simulink model "LAB2_DirectDiscreteDesign_Robust"  (R2025b)
settings: Solver=VariableStepAuto  StartTime=0.0  StopTime=2  FixedStep=T  RelTol=1e-3
values from neighbouring files (symbols this model uses):
  gamma_o = [gamma(2)-L*gamma(1), (phi22-L*phi12)*L+phi21-L*phi11]    [LAB2_2_DDD_Robust.m]
  Ho = [0;1]    [LAB2_2_DDD_Robust.m]
  Jo = [0 1; 0 L]    [LAB2_2_DDD_Robust.m]
  K = Ke(2:3)    [LAB2_2_DDD_Robust.m]
  Ki = Ke(1)    [LAB2_2_DDD_Robust.m]
  Nr = Nu + K * Nx    [LAB2_2_DDD_Robust.m]
  phi_o = lambda_o_dt    [LAB2_2_DDD_Robust.m]
  step_amplitude = 60    [LAB2_2_DDD_Robust.m]
  T = 0.2    [LAB2_2_DDD_Robust.m]
undefined symbols (not defined in the file or in its folder): DiscIntNeverNeededParam, pulse2deg
settings Model: ExtModeTrigDuration=100001  Creator=delpratogi  LastModifiedBy=Gioele
settings HardwareCC: ProdBitPerLong=64.0  ProdHWDeviceType=Intel->x86-64 (Linux 64)
settings RTWCC: SystemTargetFile=sldrt.tlc  TemplateMakefile=sldrt.tmf  RTWCompilerOptimization=on  Description=Simulink Desktop Real-Time
settings CodeAppCC: MaxIdLength=95.0
settings SimulinkDesktopRealTimeCC: ExtModeTransport=0.0  ExtModeStaticAllocSize=1000000.0  TargetLibSuffix=_sldrt.a  TargetPreCompLibLocation=C:\Program Files\MATLAB\R2025b\toolbox\sldrt\lib\win64  MultiwordLength=2048.0  DynamicStringBufferSize=256.0  ParMdlRefBuildCompliant=on  PreserveMATLABNamespacesInGeneratedCode=on  SubcomponentCodeInterfacePackaging=Reusable function  SupportVariableSizeSignals=off

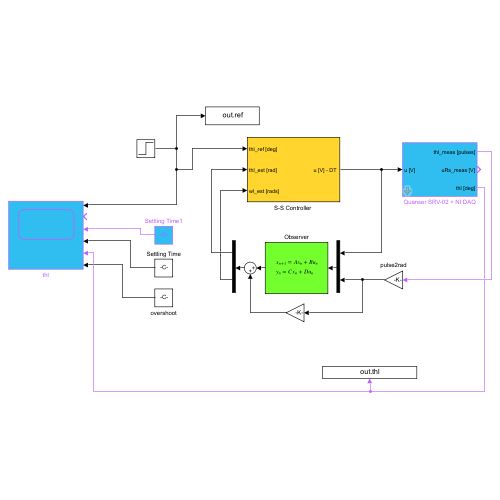
[thumbnail: Simulink's stored preview of the top-level diagram]
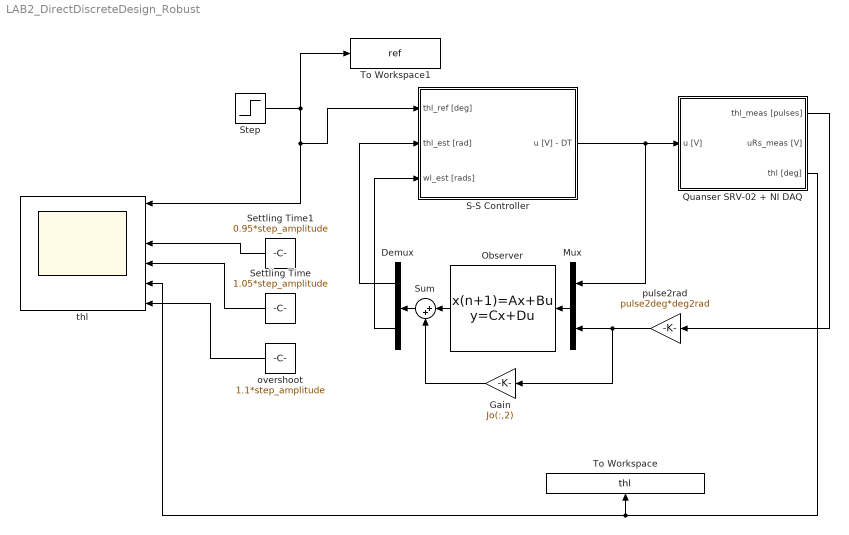
== system LAB2_DirectDiscreteDesign_Robust ==
  Demux : Demux  Outputs=2
  Gain : Gain  Gain=Jo(:,2)
  Mux : Mux  Inputs=2
  Observer : DiscreteStateSpace  A=phi_o  B=gamma_o  C=Ho  D=zeros(2,2)  SampleTime=T
  Quanser SRV-02 + NI DAQ : Subsystem  mask(Quanser SRV-02 (with inertial load) + NI DAQ){Ts=T, fricType=Coulomb + viscous}
      mask prompts: Ts "NI DAQ Sample Time:"; fricType "Friction model"
      mask help: Quanser SRV-02 (with inertial load) + NI DAQ model.
      mask init:
      | %%  Sensors data
      | 
      | %   shunt resistor
      | sens.curr.Rs = 0.5;                         %   resistance [Ohm]   
      | sens.curr.uRs_std = 0.01;                   %   voltage noise standard dev [V]                           
      | sens.curr.uRs_var = sens.curr.uRs_std^2;	%   voltage noise variance [V^2]
      | 
      | %   Hewlett-Packard HEDS-5540#A06 optical encoder
      | sens.enc.ppr = 500*4;                       %   pulses per rotation
      | sens.enc.pulse2deg = 360/sens.enc.ppr;      %   [pulses] -> [deg]
      | sens.enc.pulse2rad = 2*pi/sens.enc.ppr;     %   [pulses] -> [rad]
      | sens.enc.deg2pulse = sens.enc.ppr/360;      %   [deg] -> [pulses]
      | sens.enc.rad2pulse = sens.enc.ppr/2/pi;     %   [rad] -> [pulses]
      | 
      | 
      | %%  Data acquisition board (daq) data
      | 
      | %   NI PCI-6221 DAC data
      | daq.dac.bits = 16;                                  %   resolution (bits)
      | daq.dac.fs   = 10;                                  %   full scale 
      | daq.dac.q    = 2*daq.dac.fs/(2^daq.dac.bits-1);     %	quantization
      | 
      | %   NI PCI-6221 ADC data
      | daq.adc.bits = 16;                                  %   resolution (bits)
      | daq.adc.fs   = 10;                                  %   full scale (as set in SLDRT Analog Input block)
      | daq.adc.q    = 2*daq.adc.fs/(2^daq.adc.bits-1);     %   quantization
      mask Help:
      | Riccardo Antonello (antonello@dei.unipd.it)
      | 
      | April 24, 2020
      | 
      | Dept. of Information Engineering, University of Padova
      mask TypeOptions fricType: Coulomb + viscous | Karnopp
  "S-S Controller " : Subsystem
  Settling Time : Constant  Value=1.05*step_amplitude
  Settling Time1 : Constant  Value=0.95*step_amplitude
  Step : Step  Time=0  After=step_amplitude  ZeroCross=off
  Sum : Sum  Inputs=|++
  To Workspace : ToWorkspace  VariableName=thl  SaveFormat=Structure With Time  SampleTime=-1
  To Workspace1 : ToWorkspace  VariableName=ref  SaveFormat=Structure With Time  SampleTime=-1
  overshoot : Constant  Value=1.1*step_amplitude
  pulse2rad : Gain  Gain=pulse2deg*deg2rad
  thl : Scope  NumInputPorts=6
      settings: ActiveDisplayYMinimum=-8.2499999999999982  ActiveDisplayYMaximum=74.25
  wires:
  Demux/2 -> "S-S Controller "/3(wl_est [rads])
  "S-S Controller "/1("u [V] - DT ") -> Quanser SRV-02 + NI DAQ/1(u [V]), Mux/1
  Demux/1 -> "S-S Controller "/2(thl_est [rad])
  Mux/1 -> Observer/1
  Quanser SRV-02 + NI DAQ/1(thl_meas [pulses]) -> pulse2rad/1
  pulse2rad/1 -> Gain/1, Mux/2
  Sum/1 -> Demux/1
  Observer/1 -> Sum/1
  Gain/1 -> Sum/2
  overshoot/1 -> thl/6
  Settling Time/1 -> thl/4
  Settling Time1/1 -> thl/3
  Step/1 -> To Workspace1/1, thl/1, "S-S Controller "/1(thl_ref [deg])
  Quanser SRV-02 + NI DAQ/3(thl [deg]) -> thl/5, To Workspace/1

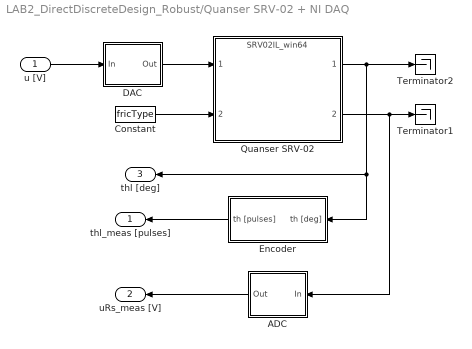
== system LAB2_DirectDiscreteDesign_Robust/Quanser SRV-02 + NI DAQ ==
  u [V] : Inport
  ADC : Subsystem
  Constant : Constant  Value=fricType
  DAC : Subsystem
  Encoder : Subsystem
  Quanser SRV-02 : ModelReference  ModelNameDialog=SRV02IL_win64.slxp  ModelReferenceVersion=1.44  CopyOfModelProtected=on
  Terminator1 : Terminator
  Terminator2 : Terminator
  thl_meas [pulses] : Outport
  uRs_meas [V] : Outport  Port=2
  thl [deg] : Outport  Port=3
  wires:
  Encoder/1(th [pulses]) -> thl_meas [pulses]/1
  ADC/1(Out) -> uRs_meas [V]/1
  DAC/1(Out) -> Quanser SRV-02/1
  Quanser SRV-02/2 -> ADC/1(In), Terminator1/1
  u [V]/1 -> DAC/1(In)
  Constant/1 -> Quanser SRV-02/2
  Quanser SRV-02/1 -> Encoder/1(th [deg]), thl [deg]/1, Terminator2/1

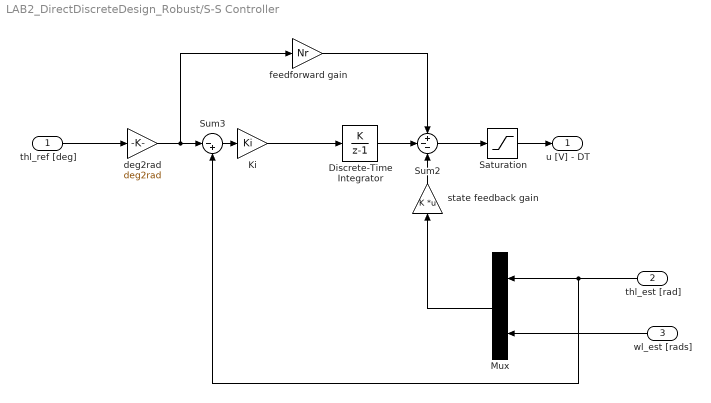
== system LAB2_DirectDiscreteDesign_Robust/S-S Controller  ==
  thl_ref [deg] : Inport
  thl_est [rad] : Inport  Port=2
  wl_est [rads] : Inport  Port=3
  " feedforward gain" : Gain  Gain=Nr
  Discrete-Time Integrator : DiscreteIntegrator  IntegratorMethod=Accumulation: Forward Euler  SampleTime=T  ICPrevOutput=DiscIntNeverNeededParam  ICPrevScaledInput=DiscIntNeverNeededParam
  Ki : Gain  Gain=Ki
  Mux : Mux  Inputs=2
  Saturation : Saturate  UpperLimit=10  LowerLimit=-10  ZeroCross=off
  Sum2 : Sum  Inputs=+--
  Sum3 : Sum  Inputs=|-+
  deg2rad : Gain  Gain=deg2rad
  state feedback gain : Gain  Gain=K  Multiplication=Matrix(K*u)
  "u [V] - DT " : Outport
  wires:
  Mux/1 -> state feedback gain/1
  deg2rad/1 -> " feedforward gain"/1, Sum3/1
  Sum2/1 -> Saturation/1
  Saturation/1 -> "u [V] - DT "/1
  thl_est [rad]/1 -> Sum3/2, Mux/1
  state feedback gain/1 -> Sum2/3
  " feedforward gain"/1 -> Sum2/1
  thl_ref [deg]/1 -> deg2rad/1
  wl_est [rads]/1 -> Mux/2
  Discrete-Time Integrator/1 -> Sum2/2
  Sum3/1 -> Ki/1
  Ki/1 -> Discrete-Time Integrator/1

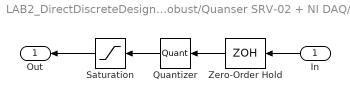
== system LAB2_DirectDiscreteDesign_Robust/Quanser SRV-02 + NI DAQ/ADC ==
  In : Inport
  Quantizer : Quantizer  QuantizationInterval=daq.adc.q
  Saturation : Saturate  UpperLimit=daq.adc.fs  LowerLimit=-daq.adc.fs
  Zero-Order Hold : ZeroOrderHold  SampleTime=Ts
  Out : Outport
  wires:
  Saturation/1 -> Out/1
  In/1 -> Zero-Order Hold/1
  Quantizer/1 -> Saturation/1
  Zero-Order Hold/1 -> Quantizer/1

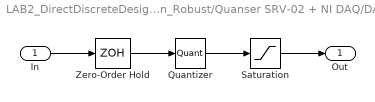
== system LAB2_DirectDiscreteDesign_Robust/Quanser SRV-02 + NI DAQ/DAC ==
  In : Inport
  Quantizer : Quantizer  QuantizationInterval=daq.dac.q
  Saturation : Saturate  UpperLimit=daq.dac.fs  LowerLimit=-daq.dac.fs
  Zero-Order Hold : ZeroOrderHold  SampleTime=T
  Out : Outport
  wires:
  Quantizer/1 -> Saturation/1
  In/1 -> Zero-Order Hold/1
  Zero-Order Hold/1 -> Quantizer/1
  Saturation/1 -> Out/1

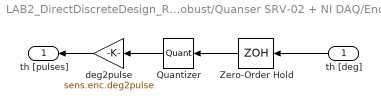
== system LAB2_DirectDiscreteDesign_Robust/Quanser SRV-02 + NI DAQ/Encoder ==
  th [deg] : Inport
  Quantizer : Quantizer  QuantizationInterval=sens.enc.pulse2deg
  Zero-Order Hold : ZeroOrderHold  SampleTime=T
  deg2pulse : Gain  Gain=sens.enc.deg2pulse
  th [pulses] : Outport
  wires:
  Quantizer/1 -> deg2pulse/1
  th [deg]/1 -> Zero-Order Hold/1
  Zero-Order Hold/1 -> Quantizer/1
  deg2pulse/1 -> th [pulses]/1
